simulink model "sampleModel162"  (Simulink 9.1)
settings: Solver=VariableStepAuto  StartTime=0.0  StopTime=10.0  RelTol=1e-3
undefined symbols (not defined in the file): DiscIntNeverNeededParam, magnitude, Newton, Raphson
libraries: simulink x49
(part 1 of 2)
settings Model: SuppressorTable="22 serialization::archive 11 0 6 0 0 2 8 0 0 0 0 6 0 0 1 0 22 sampleModel162/cfblk89 0 6 0 0 2 8 0 0 0 0 6 41 Simulink:DataType:WarningOverFlowDetected 0 0 0 6 0  0  0 0 0 0 8 20160608 0 0 0 15 23 17 0 1 40 SimulinkFixedPoint:util:Overflowoccurred 0 0 0  0  8 20160608 0 15 23 17 0 1 1 0 22 sampleModel162/cfblk90 2 8 0 41 Simulink:DataType:WarningOverFlowDetected 0 0 0  0  8 20160608 0 15 23 17 0 1 40 SimulinkFixedPoint:util:Overflowoccurred 0 0 0  0  8 20160608 0 15 23 17 0 1"  Creator=DELL  LastModifiedBy=DELL
settings DataIOCC: SaveFormat=Dataset
settings OptimizationCC: LifeSpan=auto
settings DebuggingCC: UnderspecifiedInitializationDetection=Simplified  MergeDetectMultiDrivingBlocksExec=error  SFUnexpectedBacktrackingDiag=error  SFNoUnconditionalDefaultTransitionDiag=error  SFExecutionAtInitializationDiag=warning
settings HardwareCC: ProdBitPerPointer=64  ProdBitPerSizeT=64  ProdBitPerPtrDiffT=64  ProdLargestAtomicFloat=Float  ProdIntDivRoundTo=Zero  ProdEndianess=LittleEndian  ProdWordSize=64  ProdHWDeviceType=Intel->x86-64 (Windows64)
settings ModelReferenceCC: PropagateSignalLabelsOutOfModel=on
settings CodeAppCC: StateflowObjectComments=off
settings GRTTargetCC: TargetLangStandard=C99 (ISO)  CombineOutputUpdateFcns=on  GRTInterface=off
settings ConfigComp: CovMetricSettings=dwe  CovHtmlReporting=off  CovSaveCumulativeToWorkspaceVar=off  CovSaveSingleToWorkspaceVar=off  CovExternalEMLEnable=on

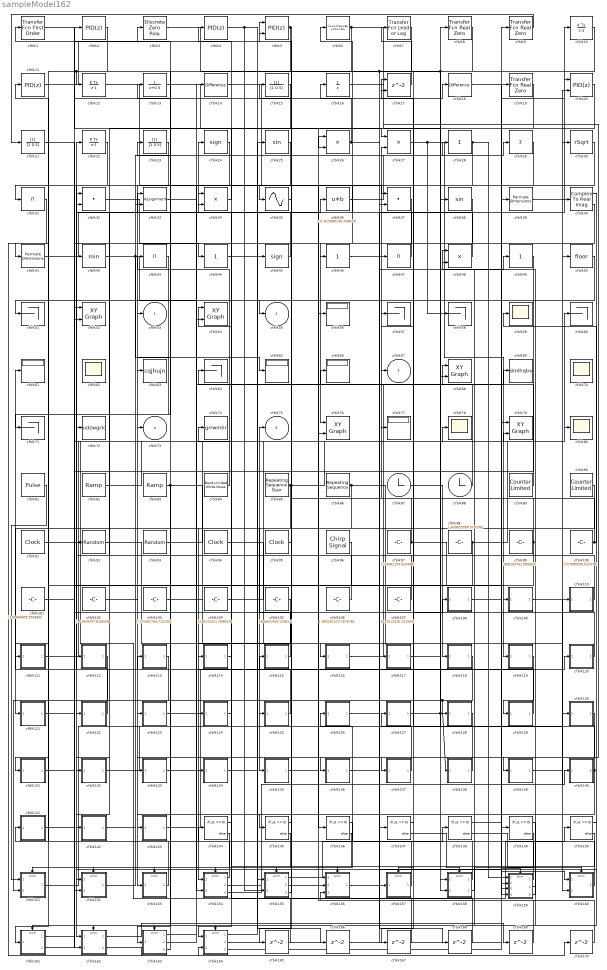
== system sampleModel162 ==
  cfblk1 : simulink/Discrete/Transfer Fcn First Order  PoleZ=0.95  ICPrevOutput=0.0  DoSatur=off
      settings: SourceProductName=Simulink
  cfblk10 : DiscreteIntegrator  ICPrevOutput=DiscIntNeverNeededParam  ICPrevScaledInput=DiscIntNeverNeededParam
  cfblk100 : Constant  Value=[727898558.012478]  SampleTime=1
  cfblk101 : Constant  Value=[149946805.550680]  SampleTime=1
  cfblk102 : Constant  Value=[-62429797.816093]  SampleTime=1
  cfblk103 : Constant  Value=[-175382764.712235]  SampleTime=1
  cfblk104 : Constant  Value=[146113221.789037]  SampleTime=1
  cfblk105 : Constant  Value=[906421434.125611]  SampleTime=1
  cfblk106 : Constant  Value=[-865261573.767678]  SampleTime=1
  cfblk107 : Constant  Value=[813312335.221064]  SampleTime=1
  cfblk108 : Subsystem
  cfblk109 : Subsystem
  cfblk11 : simulink/Continuous/PID Controller  Controller=PID  TimeDomain=Discrete-time  SampleTime=1  IntegratorMethod=Forward Euler  FilterMethod=Forward Euler  Form=Parallel  UseFilter=on  ControllerParametersSource=internal  P=1  I=1  D=0  N=100  InitialConditionSource=internal  InitialConditionForIntegrator=0  InitialConditionForFilter=0  ExternalReset=none  LimitOutput=off  UpperSaturationLimit=inf  LowerSaturationLimit=-inf  LinearizeAsGain=off  AntiWindupMode=none  Kb=1  TrackingMode=off  Kt=1  PParamMin=[]  PParamMax=[]  IParamMin=[]  IParamMax=[]  DParamMin=[]  DParamMax=[]  NParamMin=[]  NParamMax=[]  KbParamMin=[]  KbParamMax=[]  KtParamMin=[]  KtParamMax=[]  POutMin=[]  POutMax=[]  IOutMin=[]  IOutMax=[]  DOutMin=[]  DOutMax=[]  NOutMin=[]  NOutMax=[]  KbOutMin=[]  KbOutMax=[]  KtOutMin=[]  KtOutMax=[]  IntegratorOutMin=[]  IntegratorOutMax=[]  FilterOutMin=[]  FilterOutMax=[]  SumOutMin=[]  SumOutMax=[]  SumI1OutMin=[]  SumI1OutMax=[]  SumI2OutMin=[]  SumI2OutMax=[]  SumI3OutMin=[]  SumI3OutMax=[]  SumDOutMin=[]  SumDOutMax=[]  SaturationOutMin=[]  SaturationOutMax=[]  IntegratorContinuousStateAttributes=''  IntegratorStateMustResolveToSignalObject=off  IntegratorRTWStateStorageClass=Auto  FilterContinuousStateAttributes=''  FilterStateMustResolveToSignalObject=off  FilterRTWStateStorageClass=Auto  DifferentiatorICPrevScaledInput=0  DifferentiatorOutMin=[]  DifferentiatorOutMax=[]  FilterDiffOutCoefMin=[]  FilterDiffOutCoefMax=[]  SumDenOutMin=[]  SumDenOutMax=[]  SumNumOutMin=[]  SumNumOutMax=[]  ReciprocalOutMin=[]  ReciprocalOutMax=[]  DivideOutMin=[]  DivideOutMax=[]  TunerSelectOption=Transfer Function Based (PID Tuner App)
  cfblk110 : Subsystem
  cfblk111 : Subsystem
  cfblk112 : Subsystem
  cfblk113 : Subsystem
  cfblk114 : Subsystem
  cfblk115 : Subsystem
  cfblk116 : Subsystem
  cfblk117 : Subsystem
  cfblk118 : Subsystem
  cfblk119 : Subsystem
  cfblk12 : DiscreteIntegrator  ICPrevOutput=DiscIntNeverNeededParam  ICPrevScaledInput=DiscIntNeverNeededParam
  cfblk120 : Subsystem
  cfblk121 : Subsystem
  cfblk122 : Subsystem
  cfblk123 : Subsystem
  cfblk124 : Subsystem
  cfblk125 : Subsystem
  cfblk126 : Subsystem
  cfblk127 : Subsystem
  cfblk128 : Subsystem
  cfblk129 : Subsystem
  cfblk13 : DiscreteTransferFcn  SampleTime=1
  cfblk130 : Subsystem
  cfblk131 : Subsystem
  cfblk132 : Subsystem
  cfblk133 : Subsystem
  cfblk134 : Subsystem
  cfblk135 : Subsystem
  cfblk136 : Subsystem
  cfblk137 : Subsystem
  cfblk138 : Subsystem
  cfblk139 : Subsystem
  cfblk14 : simulink/Discrete/Difference  ICPrevInput=0.0  OutMin=[]  OutMax=[]  OutDataTypeStr=Inherit: Inherit via back propagation  OutDataType=fixdt(1, 16)  OutScaling=2^-10  DoSatur=off
  cfblk140 : Subsystem
  cfblk141 : Subsystem
  cfblk142 : Subsystem
  cfblk143 : Subsystem
  cfblk{144..150} (7 alike) : If  IfExpression=u1 >= 0  SampleTime=1
  cfblk15 : DiscreteFilter  SampleTime=1
  cfblk151 : Subsystem  TreatAsAtomicUnit=on
  cfblk152 : Subsystem  TreatAsAtomicUnit=on
  cfblk153 : Subsystem  TreatAsAtomicUnit=on
  cfblk154 : Subsystem  TreatAsAtomicUnit=on
  cfblk155 : Subsystem  TreatAsAtomicUnit=on
  cfblk156 : Subsystem  TreatAsAtomicUnit=on
  cfblk157 : Subsystem  TreatAsAtomicUnit=on
  cfblk158 : Subsystem  TreatAsAtomicUnit=on
  cfblk159 : Subsystem  TreatAsAtomicUnit=on
  cfblk16 : UnitDelay
  cfblk160 : Subsystem  TreatAsAtomicUnit=on
  cfblk161 : Subsystem  TreatAsAtomicUnit=on
  cfblk162 : Subsystem  TreatAsAtomicUnit=on
  cfblk163 : Subsystem  TreatAsAtomicUnit=on
  cfblk164 : Subsystem  TreatAsAtomicUnit=on
  cfblk{165..170} (6 alike) : Delay  SampleTime=1
  cfblk17 : Delay  ShowEnablePort=on  SampleTime=1
      settings: InputPortMap=u0,e6
  cfblk18 : simulink/Discrete/Difference  ICPrevInput=0.0  OutMin=[]  OutMax=[]  OutDataTypeStr=Inherit: Inherit via back propagation  OutDataType=fixdt(1, 16)  OutScaling=2^-10  DoSatur=off
  cfblk19 : simulink/Discrete/Transfer Fcn Real Zero  ZeroZ=0.75  ICPrevInput=0.0  DoSatur=off
      settings: SourceProductName=Simulink  SourceProductBaseCode=SL
  cfblk2 : simulink/Continuous/PID Controller  Controller=PID  TimeDomain=Discrete-time  SampleTime=1  IntegratorMethod=Forward Euler  FilterMethod=Forward Euler  Form=Parallel  UseFilter=on  ControllerParametersSource=internal  P=1  I=1  D=0  N=100  InitialConditionSource=internal  InitialConditionForIntegrator=0  InitialConditionForFilter=0  ExternalReset=none  LimitOutput=off  UpperSaturationLimit=inf  LowerSaturationLimit=-inf  LinearizeAsGain=off  AntiWindupMode=none  Kb=1  TrackingMode=off  Kt=1  PParamMin=[]  PParamMax=[]  IParamMin=[]  IParamMax=[]  DParamMin=[]  DParamMax=[]  NParamMin=[]  NParamMax=[]  KbParamMin=[]  KbParamMax=[]  KtParamMin=[]  KtParamMax=[]  POutMin=[]  POutMax=[]  IOutMin=[]  IOutMax=[]  DOutMin=[]  DOutMax=[]  NOutMin=[]  NOutMax=[]  KbOutMin=[]  KbOutMax=[]  KtOutMin=[]  KtOutMax=[]  IntegratorOutMin=[]  IntegratorOutMax=[]  FilterOutMin=[]  FilterOutMax=[]  SumOutMin=[]  SumOutMax=[]  SumI1OutMin=[]  SumI1OutMax=[]  SumI2OutMin=[]  SumI2OutMax=[]  SumI3OutMin=[]  SumI3OutMax=[]  SumDOutMin=[]  SumDOutMax=[]  SaturationOutMin=[]  SaturationOutMax=[]  IntegratorContinuousStateAttributes=''  IntegratorStateMustResolveToSignalObject=off  IntegratorRTWStateStorageClass=Auto  FilterContinuousStateAttributes=''  FilterStateMustResolveToSignalObject=off  FilterRTWStateStorageClass=Auto  DifferentiatorICPrevScaledInput=0  DifferentiatorOutMin=[]  DifferentiatorOutMax=[]  FilterDiffOutCoefMin=[]  FilterDiffOutCoefMax=[]  SumDenOutMin=[]  SumDenOutMax=[]  SumNumOutMin=[]  SumNumOutMax=[]  ReciprocalOutMin=[]  ReciprocalOutMax=[]  DivideOutMin=[]  DivideOutMax=[]  TunerSelectOption=Transfer Function Based (PID Tuner App)
  cfblk20 : simulink/Continuous/PID Controller (2DOF)  Controller=PID  TimeDomain=Discrete-time  SampleTime=1  IntegratorMethod=Forward Euler  FilterMethod=Forward Euler  Form=Parallel  UseFilter=on  ControllerParametersSource=internal  P=1  I=1  D=0  N=100  b=1  c=1  InitialConditionSource=internal  InitialConditionForIntegrator=0  InitialConditionForFilter=0  ExternalReset=none  LimitOutput=off  UpperSaturationLimit=inf  LowerSaturationLimit=-inf  LinearizeAsGain=off  AntiWindupMode=none  Kb=1  TrackingMode=off  Kt=1  PParamMin=[]  PParamMax=[]  IParamMin=[]  IParamMax=[]  DParamMin=[]  DParamMax=[]  NParamMin=[]  NParamMax=[]  bParamMin=[]  bParamMax=[]  cParamMin=[]  cParamMax=[]  KbParamMin=[]  KbParamMax=[]  KtParamMin=[]  KtParamMax=[]  POutMin=[]  POutMax=[]  IOutMin=[]  IOutMax=[]  DOutMin=[]  DOutMax=[]  NOutMin=[]  NOutMax=[]  bOutMin=[]  bOutMax=[]  cOutMin=[]  cOutMax=[]  KbOutMin=[]  KbOutMax=[]  KtOutMin=[]  KtOutMax=[]  IntegratorOutMin=[]  IntegratorOutMax=[]  FilterOutMin=[]  FilterOutMax=[]  SumOutMin=[]  SumOutMax=[]  Sum1OutMin=[]  Sum1OutMax=[]  Sum2OutMin=[]  Sum2OutMax=[]  Sum3OutMin=[]  Sum3OutMax=[]  SumI1OutMin=[]  SumI1OutMax=[]  SumI2OutMin=[]  SumI2OutMax=[]  SumI3OutMin=[]  SumI3OutMax=[]  SumDOutMin=[]  SumDOutMax=[]  SaturationOutMin=[]  SaturationOutMax=[]  IntegratorContinuousStateAttributes=''  IntegratorStateMustResolveToSignalObject=off  IntegratorRTWStateStorageClass=Auto  FilterContinuousStateAttributes=''  FilterStateMustResolveToSignalObject=off  FilterRTWStateStorageClass=Auto  DifferentiatorICPrevScaledInput=0  DifferentiatorOutMin=[]  DifferentiatorOutMax=[]  FilterDiffOutCoefMin=[]  FilterDiffOutCoefMax=[]  SumDenOutMin=[]  SumDenOutMax=[]  SumNumOutMin=[]  SumNumOutMax=[]  ReciprocalOutMin=[]  ReciprocalOutMax=[]  DivideOutMin=[]  DivideOutMax=[]  TunerSelectOption=Transfer Function Based (PID Tuner App)
  cfblk21 : DiscreteFilter  SampleTime=1
  cfblk22 : DiscreteIntegrator  ICPrevOutput=DiscIntNeverNeededParam  ICPrevScaledInput=DiscIntNeverNeededParam
  cfblk23 : DiscreteFilter  SampleTime=1
  cfblk24 : Signum
  cfblk25 : Trigonometry
  cfblk26 : Product  Inputs=**
  cfblk27 : Product
  cfblk{28,44,46,49} (4 alike) : simulink/Math Operations/Slider Gain  gain=1  low=0  high=2
  cfblk29 : Sum  Inputs=+
  cfblk3 : DiscreteZeroPole  Poles=[0 0.5]  Gain=1
  cfblk30 : Sqrt  Operator=rSqrt  AlgorithmType=Newton-Raphson  SaturateOnIntegerOverflow=on
  cfblk31 : Product  Inputs=*
  cfblk32 : DotProduct  InputSameDT=on  OutDataTypeStr=Inherit: Inherit via internal rule
  cfblk33 : Assignment  DiagnosticForDimensions=Warning  IndexOptions=Index vector (dialog)  Indices=1  OutputSizes=1
  cfblk34 : Product  Inputs=**
  cfblk35 : Sin  TimeSource=Use external signal  SampleTime=0
  cfblk36 : Bias  Bias=[-815080136.708875]
  cfblk37 : DotProduct  InputSameDT=on  OutDataTypeStr=Inherit: Inherit via internal rule
  cfblk38 : Trigonometry
  cfblk39 : PermuteDimensions
  cfblk4 : simulink/Continuous/PID Controller  Controller=PID  TimeDomain=Discrete-time  SampleTime=1  IntegratorMethod=Forward Euler  FilterMethod=Forward Euler  Form=Parallel  UseFilter=on  ControllerParametersSource=internal  P=1  I=1  D=0  N=100  InitialConditionSource=internal  InitialConditionForIntegrator=0  InitialConditionForFilter=0  ExternalReset=none  LimitOutput=off  UpperSaturationLimit=inf  LowerSaturationLimit=-inf  LinearizeAsGain=off  AntiWindupMode=none  Kb=1  TrackingMode=off  Kt=1  PParamMin=[]  PParamMax=[]  IParamMin=[]  IParamMax=[]  DParamMin=[]  DParamMax=[]  NParamMin=[]  NParamMax=[]  KbParamMin=[]  KbParamMax=[]  KtParamMin=[]  KtParamMax=[]  POutMin=[]  POutMax=[]  IOutMin=[]  IOutMax=[]  DOutMin=[]  DOutMax=[]  NOutMin=[]  NOutMax=[]  KbOutMin=[]  KbOutMax=[]  KtOutMin=[]  KtOutMax=[]  IntegratorOutMin=[]  IntegratorOutMax=[]  FilterOutMin=[]  FilterOutMax=[]  SumOutMin=[]  SumOutMax=[]  SumI1OutMin=[]  SumI1OutMax=[]  SumI2OutMin=[]  SumI2OutMax=[]  SumI3OutMin=[]  SumI3OutMax=[]  SumDOutMin=[]  SumDOutMax=[]  SaturationOutMin=[]  SaturationOutMax=[]  IntegratorContinuousStateAttributes=''  IntegratorStateMustResolveToSignalObject=off  IntegratorRTWStateStorageClass=Auto  FilterContinuousStateAttributes=''  FilterStateMustResolveToSignalObject=off  FilterRTWStateStorageClass=Auto  DifferentiatorICPrevScaledInput=0  DifferentiatorOutMin=[]  DifferentiatorOutMax=[]  FilterDiffOutCoefMin=[]  FilterDiffOutCoefMax=[]  SumDenOutMin=[]  SumDenOutMax=[]  SumNumOutMin=[]  SumNumOutMax=[]  ReciprocalOutMin=[]  ReciprocalOutMax=[]  DivideOutMin=[]  DivideOutMax=[]  TunerSelectOption=Transfer Function Based (PID Tuner App)
  cfblk40 : ComplexToRealImag
  cfblk41 : PermuteDimensions
  cfblk42 : MinMax
  cfblk43 : Product  Inputs=*
  cfblk45 : Signum
  cfblk47 : Product  Inputs=*
  cfblk48 : Product
  cfblk5 : simulink/Continuous/PID Controller (2DOF)  Controller=PID  TimeDomain=Discrete-time  SampleTime=1  IntegratorMethod=Forward Euler  FilterMethod=Forward Euler  Form=Parallel  UseFilter=on  ControllerParametersSource=internal  P=1  I=1  D=0  N=100  b=1  c=1  InitialConditionSource=internal  InitialConditionForIntegrator=0  InitialConditionForFilter=0  ExternalReset=none  LimitOutput=off  UpperSaturationLimit=inf  LowerSaturationLimit=-inf  LinearizeAsGain=off  AntiWindupMode=none  Kb=1  TrackingMode=off  Kt=1  PParamMin=[]  PParamMax=[]  IParamMin=[]  IParamMax=[]  DParamMin=[]  DParamMax=[]  NParamMin=[]  NParamMax=[]  bParamMin=[]  bParamMax=[]  cParamMin=[]  cParamMax=[]  KbParamMin=[]  KbParamMax=[]  KtParamMin=[]  KtParamMax=[]  POutMin=[]  POutMax=[]  IOutMin=[]  IOutMax=[]  DOutMin=[]  DOutMax=[]  NOutMin=[]  NOutMax=[]  bOutMin=[]  bOutMax=[]  cOutMin=[]  cOutMax=[]  KbOutMin=[]  KbOutMax=[]  KtOutMin=[]  KtOutMax=[]  IntegratorOutMin=[]  IntegratorOutMax=[]  FilterOutMin=[]  FilterOutMax=[]  SumOutMin=[]  SumOutMax=[]  Sum1OutMin=[]  Sum1OutMax=[]  Sum2OutMin=[]  Sum2OutMax=[]  Sum3OutMin=[]  Sum3OutMax=[]  SumI1OutMin=[]  SumI1OutMax=[]  SumI2OutMin=[]  SumI2OutMax=[]  SumI3OutMin=[]  SumI3OutMax=[]  SumDOutMin=[]  SumDOutMax=[]  SaturationOutMin=[]  SaturationOutMax=[]  IntegratorContinuousStateAttributes=''  IntegratorStateMustResolveToSignalObject=off  IntegratorRTWStateStorageClass=Auto  FilterContinuousStateAttributes=''  FilterStateMustResolveToSignalObject=off  FilterRTWStateStorageClass=Auto  DifferentiatorICPrevScaledInput=0  DifferentiatorOutMin=[]  DifferentiatorOutMax=[]  FilterDiffOutCoefMin=[]  FilterDiffOutCoefMax=[]  SumDenOutMin=[]  SumDenOutMax=[]  SumNumOutMin=[]  SumNumOutMax=[]  ReciprocalOutMin=[]  ReciprocalOutMax=[]  DivideOutMin=[]  DivideOutMax=[]  TunerSelectOption=Transfer Function Based (PID Tuner App)
  cfblk50 : Rounding
  cfblk{51,57..58,60,64,71} (6 alike) : Terminator
  cfblk{52,54,68,76,79} (5 alike) : simulink/Sinks/XY Graph  xmin=-1  xmax=1  ymin=-1  ymax=1  st=-1
  cfblk{56,61,65..66,77} (5 alike) : Display
  cfblk{59,62,70,78,80} (5 alike) : Scope
      cfblk62 settings: Floating=on
      cfblk70 settings: Floating=on
  cfblk6 : DiscreteStateSpace
  cfblk63 : ToWorkspace  VariableName=cqjhujn  SaveFormat=Timeseries  SampleTime=-1
  cfblk69 : ToWorkspace  VariableName=dmlhqbv  SaveFormat=Timeseries  SampleTime=-1
  cfblk7 : simulink/Discrete/Transfer Fcn Lead or Lag  PoleZ=0.95  ZeroZ=0.75  ICPrevOutput=0.0  ICPrevInput=0.0  DoSatur=off
      settings: SourceProductName=Simulink  SourceProductBaseCode=SL
  cfblk72 : ToWorkspace  VariableName=udzwgck  SaveFormat=Timeseries  SampleTime=-1
  cfblk74 : ToWorkspace  VariableName=grrwmhr  SaveFormat=Timeseries  SampleTime=-1
  cfblk8 : simulink/Discrete/Transfer Fcn Real Zero  ZeroZ=0.75  ICPrevInput=0.0  DoSatur=off
      settings: SourceProductName=Simulink  SourceProductBaseCode=SL
  cfblk81 : DiscretePulseGenerator  PulseType=Time based  Amplitude=[-1371846.449111]  Period=[72395569.989002]  PulseWidth=5  PhaseDelay=[9.000000]
  cfblk82 : simulink/Sources/Ramp  slope=[5140.421484]  start=[47.590381]  InitialOutput=[-206299.463391]
  cfblk83 : simulink/Sources/Ramp  slope=[-8341.390196]  start=[43.939396]  InitialOutput=[-754794.637201]
  cfblk84 : simulink/Sources/Band-Limited White Noise  Cov=[7560464618.662546]  Ts=0.1  seed=[9065001128.000000]
  cfblk85 : simulink/Sources/Repeating Sequence Stair  OutValues=[-79011152.103958, -456733271.397849]  tsamp=-1  OutMin=[]  OutMax=[]  OutDataTypeStr=double  OutputDataTypeScalingMode=double  OutDataType=fixdt(0,8)  ConRadixGroup=Best Precision: Vector-wise  OutScaling=2^-12
  cfblk86 : simulink/Sources/Repeating Sequence  rep_seq_t=[0 2]  rep_seq_y=[-862919646.627076, -121342680.384582]
  cfblk87 : Clock
  cfblk88 : Clock
  cfblk89 : simulink/Sources/Counter Limited  uplimit=[824.000000]  tsamp=-1
  cfblk9 : simulink/Discrete/Transfer Fcn Real Zero  ZeroZ=0.75  ICPrevInput=0.0  DoSatur=off
      settings: SourceProductName=Simulink  SourceProductBaseCode=SL
  cfblk90 : simulink/Sources/Counter Limited  uplimit=[298.000000]  tsamp=-1
  cfblk91 : DigitalClock
  cfblk92 : RandomNumber  Mean=[-60678.124830]  Variance=[62859.906878]  Seed=[18431920.000000]  SampleTime=0.1
  cfblk93 : UniformRandomNumber  Minimum=[-2959977652.124598]  Maximum=[440301292.630647]  Seed=[41048107.000000]  SampleTime=0.1
  cfblk94 : DigitalClock
  cfblk95 : DigitalClock
  cfblk96 : simulink/Sources/Chirp Signal  f1=[-414625876.542801]  T=[476939218.482737]  f2=[-707117522.097986]
  cfblk97 : Constant  Value=[174581154.924498]  SampleTime=1
  cfblk98 : Constant  Value=[-639855958.573706]  SampleTime=1
  cfblk99 : Constant  Value=[965265761.586653]  SampleTime=1
  cfblk53 : Outport
  cfblk55 : Outport  Port=2
  cfblk67 : Outport  Port=3
  cfblk73 : Outport  Port=4
  cfblk75 : Outport  Port=5
  wires:
  cfblk23/1 -> cfblk153/1(cfblk1)
  cfblk84/1 -> cfblk1/1
  cfblk91/1 -> cfblk150/1, cfblk79/2
  cfblk90/1 -> cfblk154/1(cfblk1)
  cfblk114/1(cfblk2) -> cfblk164/1(cfblk1)
  cfblk41/1 -> cfblk33/1
  cfblk155/1(cfblk2) -> cfblk148/1
  cfblk112/1(cfblk2) -> cfblk162/1(cfblk1)
  cfblk11/1 -> cfblk5/1
  cfblk110/1(cfblk2) -> cfblk22/1
  cfblk50/1 -> cfblk51/1
  cfblk116/1(cfblk2) -> cfblk68/1
  cfblk100/1 -> cfblk59/1, cfblk77/1
  cfblk13/1 -> cfblk27/1
  cfblk36/1 -> cfblk29/1
  cfblk6/1 -> cfblk139/1(cfblk1), cfblk35/1
  cfblk24/1 -> cfblk63/1
  cfblk115/1(cfblk2) -> cfblk75/1
  cfblk94/1 -> cfblk116/1(cfblk1)
  cfblk48/1 -> cfblk24/1
  cfblk86/1 -> cfblk121/1(cfblk1), cfblk158/2(cfblk16)
  cfblk119/1(cfblk2) -> cfblk129/1(cfblk1)
  cfblk25/1 -> cfblk122/1(cfblk1)
  cfblk39/1 -> cfblk10/1
  cfblk140/1(cfblk2) -> cfblk143/1(cfblk1), cfblk17/2
  cfblk105/1 -> cfblk114/1(cfblk1)
  cfblk12/1 -> cfblk146/1
  cfblk81/1 -> cfblk151/1(cfblk1)
  cfblk82/1 -> cfblk14/1
  cfblk129/1(cfblk2) -> cfblk61/1
  cfblk99/1 -> cfblk27/2, cfblk131/1(cfblk1)
  cfblk38/1 -> cfblk76/1
  cfblk85/1 -> cfblk145/1, cfblk47/1, cfblk135/1(cfblk1)
  cfblk20/1 -> cfblk73/1
  cfblk122/1(cfblk2) -> cfblk72/1
  cfblk101/1 -> cfblk2/1
  cfblk14/1 -> cfblk37/1
  cfblk27/1 -> cfblk119/1(cfblk1), cfblk58/1
  cfblk37/1 -> cfblk42/1
  cfblk102/1 -> cfblk123/1(cfblk1)
  cfblk10/1 -> cfblk137/1(cfblk1), cfblk68/2
  cfblk160/1(cfblk2) -> cfblk126/1(cfblk1)
  cfblk133/1(cfblk2) -> cfblk26/1
  cfblk43/1 -> cfblk71/1
  cfblk26/1 -> cfblk16/1, cfblk159/2(cfblk8)
  cfblk97/1 -> cfblk149/1, cfblk5/2
  cfblk123/1(cfblk2) -> cfblk120/1(cfblk1)
  cfblk151/1(cfblk2) -> cfblk110/1(cfblk1)
  cfblk44/1 -> cfblk45/1
  cfblk87/1 -> cfblk118/1(cfblk1)
  cfblk21/1 -> cfblk109/1(cfblk1)
  cfblk4/1 -> cfblk155/2(cfblk14), cfblk166/1
  cfblk135/1(cfblk2) -> cfblk56/1
  cfblk98/1 -> cfblk60/1, cfblk134/1(cfblk1)
  cfblk88/1 -> cfblk64/1
  cfblk152/1(cfblk2) -> cfblk36/1
  cfblk89/1 -> cfblk67/1
  cfblk158/1(cfblk2) -> cfblk34/1
  cfblk153/1(cfblk2) -> cfblk141/1(cfblk1)
  cfblk96/1 -> cfblk161/1(cfblk1)
  cfblk103/1 -> cfblk157/1(cfblk1)
  cfblk8/1 -> cfblk37/2, cfblk125/1(cfblk1)
  cfblk95/1 -> cfblk15/1
  cfblk93/1 -> cfblk19/1
  cfblk113/1(cfblk2) -> cfblk132/1(cfblk1)
  cfblk137/1(cfblk2) -> cfblk127/1(cfblk1)
  cfblk15/1 -> cfblk124/1(cfblk1)
  cfblk29/1 -> cfblk154/2(cfblk7)
  cfblk32/1 -> cfblk44/1
  cfblk134/1(cfblk2) -> cfblk69/1
  cfblk124/1(cfblk2) -> cfblk54/1
  cfblk138/1(cfblk2) -> cfblk136/1(cfblk1)
  cfblk49/1 -> cfblk162/2(cfblk12)
  cfblk121/1(cfblk2) -> cfblk78/1
  cfblk163/1(cfblk2) -> cfblk66/1
  cfblk42/1 -> cfblk54/2, cfblk65/1
  cfblk30/1 -> cfblk46/1
  cfblk19/1 -> cfblk142/1(cfblk1)
  cfblk161/1(cfblk2) -> cfblk108/1(cfblk1)
  cfblk120/1(cfblk2) -> cfblk57/1
  cfblk9/1 -> cfblk21/1
  cfblk28/1 -> cfblk111/1(cfblk1), cfblk159/1(cfblk1)
  cfblk142/1(cfblk2) -> cfblk28/1
  cfblk7/1 -> cfblk31/1
  cfblk3/1 -> cfblk38/1
  cfblk108/1(cfblk2) -> cfblk20/1
  cfblk33/1 -> cfblk17/1
  cfblk136/1(cfblk2) -> cfblk49/1
  cfblk117/1(cfblk2) -> cfblk80/1
  cfblk118/1(cfblk2) -> cfblk151/2(cfblk14), cfblk128/1(cfblk1)
  cfblk31/1 -> cfblk164/2(cfblk10)
  cfblk154/1(cfblk2) -> cfblk113/1(cfblk1)
  cfblk47/1 -> cfblk6/1
  cfblk35/1 -> cfblk55/1
  cfblk132/1(cfblk2) -> cfblk9/1
  cfblk104/1 -> cfblk30/1
  cfblk45/1 -> cfblk23/1
  cfblk143/1(cfblk2) -> cfblk8/1
  cfblk141/1(cfblk2) -> cfblk3/1
  cfblk157/1(cfblk2) -> cfblk11/1
  cfblk109/1(cfblk2) -> cfblk130/1(cfblk1)
  cfblk156/1(cfblk2) -> cfblk40/1
  cfblk106/1 -> cfblk13/1
  cfblk127/1(cfblk2) -> cfblk138/1(cfblk1), cfblk159/3(cfblk9)
  cfblk1/1 -> cfblk26/2
  cfblk17/1 -> cfblk7/1
  cfblk128/1(cfblk2) -> cfblk163/1(cfblk1)
  cfblk161/2(cfblk8) -> cfblk52/1
  cfblk164/1(cfblk2) -> cfblk25/1
  cfblk34/1 -> cfblk4/1
  cfblk2/1 -> cfblk12/1, cfblk41/1
  cfblk5/1 -> cfblk53/1, cfblk165/1
  cfblk154/2(cfblk8) -> cfblk50/1
  cfblk164/2(cfblk11) -> cfblk79/1
  cfblk155/2(cfblk15) -> cfblk140/1(cfblk1)
  cfblk83/1 -> cfblk133/1(cfblk1), cfblk159/4(cfblk10)
  cfblk131/1(cfblk2) -> cfblk18/1
  cfblk154/3(cfblk9) -> cfblk76/2
  cfblk40/1 -> cfblk152/1(cfblk1)
  cfblk18/1 -> cfblk160/1(cfblk1)
  cfblk92/1 -> cfblk160/2(cfblk8)
  cfblk158/2(cfblk17) -> cfblk48/1
  cfblk16/1 -> cfblk158/1(cfblk1)
  cfblk164/3(cfblk12) -> cfblk39/1
  cfblk40/2 -> cfblk152/2(cfblk8)
  cfblk155/3(cfblk16) -> cfblk32/1
  cfblk107/1 -> cfblk32/2
  cfblk46/1 -> cfblk117/1(cfblk1)
  cfblk22/1 -> cfblk52/2
  cfblk139/1(cfblk2) -> cfblk20/2
  cfblk163/2(cfblk6) -> cfblk115/1(cfblk1)
  cfblk111/1(cfblk2) -> cfblk33/2
  cfblk125/1(cfblk2) -> cfblk112/1(cfblk1)
  cfblk159/1(cfblk2) -> cfblk74/1
  cfblk159/2(cfblk11) -> cfblk48/2
  cfblk159/3(cfblk12) -> cfblk144/1
  cfblk163/3(cfblk7) -> cfblk43/1
  cfblk144/1 -> cfblk151/Action
  cfblk144/2 -> cfblk152/Action
  cfblk145/1 -> cfblk153/Action
  cfblk145/2 -> cfblk154/Action
  cfblk146/1 -> cfblk155/Action
  cfblk146/2 -> cfblk156/Action
  cfblk147/1 -> cfblk157/Action
  cfblk147/2 -> cfblk158/Action
  cfblk148/1 -> cfblk159/Action
  cfblk148/2 -> cfblk160/Action
  cfblk149/1 -> cfblk161/Action
  cfblk149/2 -> cfblk162/Action
  cfblk150/1 -> cfblk163/Action
  cfblk150/2 -> cfblk164/Action
  cfblk165/1 -> cfblk34/2
  cfblk166/1 -> cfblk147/1
  cfblk130/1(cfblk2) -> cfblk167/1
  cfblk167/1 -> cfblk155/1(cfblk1)
  cfblk126/1(cfblk2) -> cfblk168/1
  cfblk168/1 -> cfblk156/1(cfblk1)
  cfblk162/1(cfblk2) -> cfblk169/1
  cfblk169/1 -> cfblk156/2(cfblk7)
  cfblk162/2(cfblk13) -> cfblk170/1
  cfblk170/1 -> cfblk156/3(cfblk8)

== system sampleModel162/cfblk108 ==
  cfblk1 : Inport
  cfblk2 : Outport
  wires:
  cfblk1/1 -> cfblk2/1

== system sampleModel162/cfblk109 ==
  cfblk1 : Inport
  cfblk2 : Outport
  wires:
  cfblk1/1 -> cfblk2/1

== system sampleModel162/cfblk110 ==
  cfblk1 : Inport
  cfblk2 : Outport
  wires:
  cfblk1/1 -> cfblk2/1

== system sampleModel162/cfblk111 ==
  cfblk1 : Inport
  cfblk2 : Outport
  wires:
  cfblk1/1 -> cfblk2/1

== system sampleModel162/cfblk112 ==
  cfblk1 : Inport
  cfblk2 : Outport
  wires:
  cfblk1/1 -> cfblk2/1

== system sampleModel162/cfblk113 ==
  cfblk1 : Inport
  cfblk2 : Outport
  wires:
  cfblk1/1 -> cfblk2/1

== system sampleModel162/cfblk114 ==
  cfblk1 : Inport
  cfblk2 : Outport
  wires:
  cfblk1/1 -> cfblk2/1

== system sampleModel162/cfblk115 ==
  cfblk1 : Inport
  cfblk2 : Outport
  wires:
  cfblk1/1 -> cfblk2/1

== system sampleModel162/cfblk116 ==
  cfblk1 : Inport
  cfblk2 : Outport
  wires:
  cfblk1/1 -> cfblk2/1

== system sampleModel162/cfblk117 ==
  cfblk1 : Inport
  cfblk2 : Outport
  wires:
  cfblk1/1 -> cfblk2/1

== system sampleModel162/cfblk118 ==
  cfblk1 : Inport
  cfblk2 : Outport
  wires:
  cfblk1/1 -> cfblk2/1

== system sampleModel162/cfblk119 ==
  cfblk1 : Inport
  cfblk2 : Outport
  wires:
  cfblk1/1 -> cfblk2/1

== system sampleModel162/cfblk120 ==
  cfblk1 : Inport
  cfblk2 : Outport
  wires:
  cfblk1/1 -> cfblk2/1

== system sampleModel162/cfblk121 ==
  cfblk1 : Inport
  cfblk2 : Outport
  wires:
  cfblk1/1 -> cfblk2/1

== system sampleModel162/cfblk122 ==
  cfblk1 : Inport
  cfblk2 : Outport
  wires:
  cfblk1/1 -> cfblk2/1

== system sampleModel162/cfblk123 ==
  cfblk1 : Inport
  cfblk2 : Outport
  wires:
  cfblk1/1 -> cfblk2/1

== system sampleModel162/cfblk124 ==
  cfblk1 : Inport
  cfblk2 : Outport
  wires:
  cfblk1/1 -> cfblk2/1

== system sampleModel162/cfblk125 ==
  cfblk1 : Inport
  cfblk2 : Outport
  wires:
  cfblk1/1 -> cfblk2/1

== system sampleModel162/cfblk126 ==
  cfblk1 : Inport
  cfblk2 : Outport
  wires:
  cfblk1/1 -> cfblk2/1

== system sampleModel162/cfblk127 ==
  cfblk1 : Inport
  cfblk2 : Outport
  wires:
  cfblk1/1 -> cfblk2/1

== system sampleModel162/cfblk128 ==
  cfblk1 : Inport
  cfblk2 : Outport
  wires:
  cfblk1/1 -> cfblk2/1

== system sampleModel162/cfblk129 ==
  cfblk1 : Inport
  cfblk2 : Outport
  wires:
  cfblk1/1 -> cfblk2/1

== system sampleModel162/cfblk130 ==
  cfblk1 : Inport
  cfblk2 : Outport
  wires:
  cfblk1/1 -> cfblk2/1

== system sampleModel162/cfblk131 ==
  cfblk1 : Inport
  cfblk2 : Outport
  wires:
  cfblk1/1 -> cfblk2/1

== system sampleModel162/cfblk132 ==
  cfblk1 : Inport
  cfblk2 : Outport
  wires:
  cfblk1/1 -> cfblk2/1

== system sampleModel162/cfblk133 ==
  cfblk1 : Inport
  cfblk2 : Outport
  wires:
  cfblk1/1 -> cfblk2/1

== system sampleModel162/cfblk134 ==
  cfblk1 : Inport
  cfblk2 : Outport
  wires:
  cfblk1/1 -> cfblk2/1

== system sampleModel162/cfblk135 ==
  cfblk1 : Inport
  cfblk2 : Outport
  wires:
  cfblk1/1 -> cfblk2/1

== system sampleModel162/cfblk136 ==
  cfblk1 : Inport
  cfblk2 : Outport
  wires:
  cfblk1/1 -> cfblk2/1

== system sampleModel162/cfblk137 ==
  cfblk1 : Inport
  cfblk2 : Outport
  wires:
  cfblk1/1 -> cfblk2/1

== system sampleModel162/cfblk138 ==
  cfblk1 : Inport
  cfblk2 : Outport
  wires:
  cfblk1/1 -> cfblk2/1

== system sampleModel162/cfblk139 ==
  cfblk1 : Inport
  cfblk2 : Outport
  wires:
  cfblk1/1 -> cfblk2/1

== system sampleModel162/cfblk140 ==
  cfblk1 : Inport
  cfblk2 : Outport
  wires:
  cfblk1/1 -> cfblk2/1

== system sampleModel162/cfblk141 ==
  cfblk1 : Inport
  cfblk2 : Outport
  wires:
  cfblk1/1 -> cfblk2/1

== system sampleModel162/cfblk142 ==
  cfblk1 : Inport
  cfblk2 : Outport
  wires:
  cfblk1/1 -> cfblk2/1

== system sampleModel162/cfblk143 ==
  cfblk1 : Inport
  cfblk2 : Outport
  wires:
  cfblk1/1 -> cfblk2/1

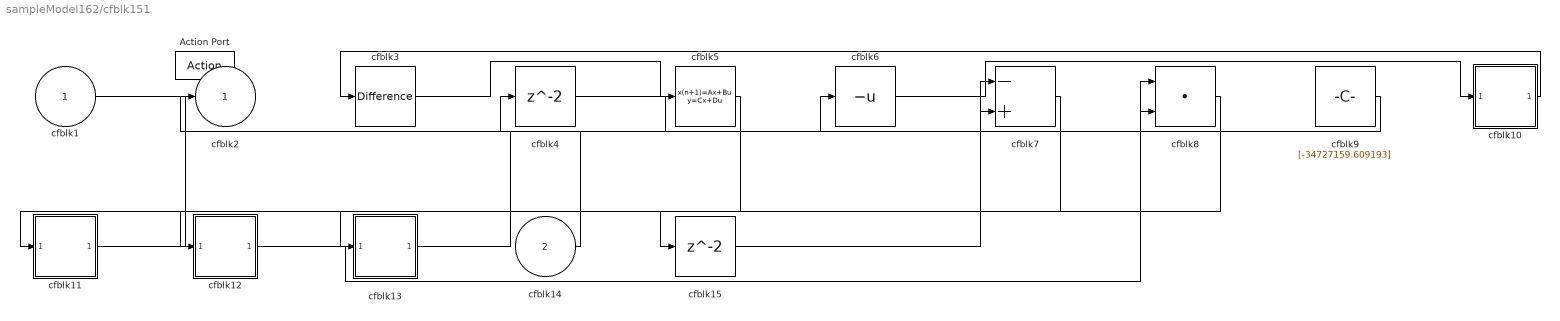
== system sampleModel162/cfblk151 ==
  cfblk1 : Inport
  cfblk14 : Inport  Port=2
  Action Port : ActionPort  ActionType=then
  cfblk10 : Subsystem
  cfblk11 : Subsystem
  cfblk12 : Subsystem
  cfblk13 : Subsystem
  cfblk15 : Delay
  cfblk3 : simulink/Discrete/Difference  ICPrevInput=0.0  OutMin=[]  OutMax=[]  OutDataTypeStr=Inherit: Inherit via back propagation  OutDataType=fixdt(1, 16)  OutScaling=2^-10  DoSatur=off
  cfblk4 : Delay
  cfblk5 : DiscreteStateSpace  SampleTime=-1
  cfblk6 : UnaryMinus
  cfblk7 : Sum  Inputs=-+
  cfblk8 : DotProduct  InputSameDT=on  OutDataTypeStr=Inherit: Inherit via internal rule
  cfblk9 : Constant  Value=[-34727159.609193]  SampleTime=1
  cfblk2 : Outport
  wires:
  cfblk5/1 -> cfblk11/1(cfblk1)
  cfblk6/1 -> cfblk10/1(cfblk1)
  cfblk14/1 -> cfblk4/1
  cfblk10/1(cfblk2) -> cfblk3/1
  cfblk12/1(cfblk2) -> cfblk8/1
  cfblk1/1 -> cfblk13/1(cfblk1)
  cfblk13/1(cfblk2) -> cfblk6/1
  cfblk11/1(cfblk2) -> cfblk7/1
  cfblk7/1 -> cfblk12/1(cfblk1)
  cfblk4/1 -> cfblk8/2
  cfblk3/1 -> cfblk5/1
  cfblk9/1 -> cfblk2/1
  cfblk8/1 -> cfblk15/1
  cfblk15/1 -> cfblk7/2

== system sampleModel162/cfblk152 ==
  cfblk1 : Inport
  cfblk8 : Inport  Port=2
  Action Port : ActionPort  ActionType=else
  cfblk3 : DiscreteIntegrator  SampleTime=-1  ICPrevOutput=DiscIntNeverNeededParam  ICPrevScaledInput=DiscIntNeverNeededParam
  cfblk4 : Gain  Gain=[981288571.279234]
  cfblk5 : Constant  Value=[52814938.085575]  SampleTime=1
  cfblk6 : Subsystem
  cfblk7 : Subsystem
  cfblk9 : Delay
  cfblk2 : Outport
  wires:
  cfblk1/1 -> cfblk3/1
  cfblk5/1 -> cfblk2/1
  cfblk4/1 -> cfblk6/1(cfblk1)
  cfblk8/1 -> cfblk7/1(cfblk1)
  cfblk6/1(cfblk2) -> cfblk9/1
  cfblk9/1 -> cfblk4/1

== system sampleModel162/cfblk153 ==
  cfblk1 : Inport
  Action Port : ActionPort  ActionType=then
  cfblk3 : DiscreteZeroPole  Poles=[0 0.5]  Gain=1  SampleTime=-1
  cfblk4 : MinMax  Function=max
  cfblk5 : Sqrt  SaturateOnIntegerOverflow=on
  cfblk6 : Constant  Value=[721223764.128831]  SampleTime=1
  cfblk7 : Constant  Value=[842996176.805068]  SampleTime=1
  cfblk8 : Subsystem
  cfblk9 : Subsystem
  cfblk2 : Outport
  wires:
  cfblk6/1 -> cfblk9/1(cfblk1)
  cfblk9/1(cfblk2) -> cfblk5/1
  cfblk5/1 -> cfblk2/1
  cfblk4/1 -> cfblk8/1(cfblk1)
  cfblk7/1 -> cfblk4/1
  cfblk1/1 -> cfblk3/1

== system sampleModel162/cfblk154 ==
  cfblk1 : Inport
  cfblk7 : Inport  Port=2
  Action Port : ActionPort  ActionType=else
  cfblk10 : DataTypeConversion
  cfblk3 : simulink/Continuous/PID Controller (2DOF)  Controller=PID  TimeDomain=Discrete-time  SampleTime=-1  IntegratorMethod=Forward Euler  FilterMethod=Forward Euler  Form=Parallel  UseFilter=on  ControllerParametersSource=internal  P=1  I=1  D=0  N=100  b=1  c=1  InitialConditionSource=internal  InitialConditionForIntegrator=0  InitialConditionForFilter=0  ExternalReset=none  LimitOutput=off  UpperSaturationLimit=inf  LowerSaturationLimit=-inf  LinearizeAsGain=off  AntiWindupMode=none  Kb=1  TrackingMode=off  Kt=1  PParamMin=[]  PParamMax=[]  IParamMin=[]  IParamMax=[]  DParamMin=[]  DParamMax=[]  NParamMin=[]  NParamMax=[]  bParamMin=[]  bParamMax=[]  cParamMin=[]  cParamMax=[]  KbParamMin=[]  KbParamMax=[]  KtParamMin=[]  KtParamMax=[]  POutMin=[]  POutMax=[]  IOutMin=[]  IOutMax=[]  DOutMin=[]  DOutMax=[]  NOutMin=[]  NOutMax=[]  bOutMin=[]  bOutMax=[]  cOutMin=[]  cOutMax=[]  KbOutMin=[]  KbOutMax=[]  KtOutMin=[]  KtOutMax=[]  IntegratorOutMin=[]  IntegratorOutMax=[]  FilterOutMin=[]  FilterOutMax=[]  SumOutMin=[]  SumOutMax=[]  Sum1OutMin=[]  Sum1OutMax=[]  Sum2OutMin=[]  Sum2OutMax=[]  Sum3OutMin=[]  Sum3OutMax=[]  SumI1OutMin=[]  SumI1OutMax=[]  SumI2OutMin=[]  SumI2OutMax=[]  SumI3OutMin=[]  SumI3OutMax=[]  SumDOutMin=[]  SumDOutMax=[]  SaturationOutMin=[]  SaturationOutMax=[]  IntegratorContinuousStateAttributes=''  IntegratorStateMustResolveToSignalObject=off  IntegratorRTWStateStorageClass=Auto  FilterContinuousStateAttributes=''  FilterStateMustResolveToSignalObject=off  FilterRTWStateStorageClass=Auto  DifferentiatorICPrevScaledInput=0  DifferentiatorOutMin=[]  DifferentiatorOutMax=[]  FilterDiffOutCoefMin=[]  FilterDiffOutCoefMax=[]  SumDenOutMin=[]  SumDenOutMax=[]  SumNumOutMin=[]  SumNumOutMax=[]  ReciprocalOutMin=[]  ReciprocalOutMax=[]  DivideOutMin=[]  DivideOutMax=[]  TunerSelectOption=Transfer Function Based (PID Tuner App)
  cfblk4 : Sin  TimeSource=Use external signal  SampleTime=0
  cfblk5 : Subsystem
  cfblk6 : Subsystem
  cfblk2 : Outport
  cfblk8 : Outport  Port=2
  cfblk9 : Outport  Port=3
  wires:
  cfblk7/1 -> cfblk2/1, cfblk3/2
  cfblk4/1 -> cfblk5/1(cfblk1)
  cfblk5/1(cfblk2) -> cfblk8/1, cfblk3/1
  cfblk3/1 -> cfblk6/1(cfblk1)
  cfblk6/1(cfblk2) -> cfblk9/1
  cfblk1/1 -> cfblk10/1
  cfblk10/1 -> cfblk4/1

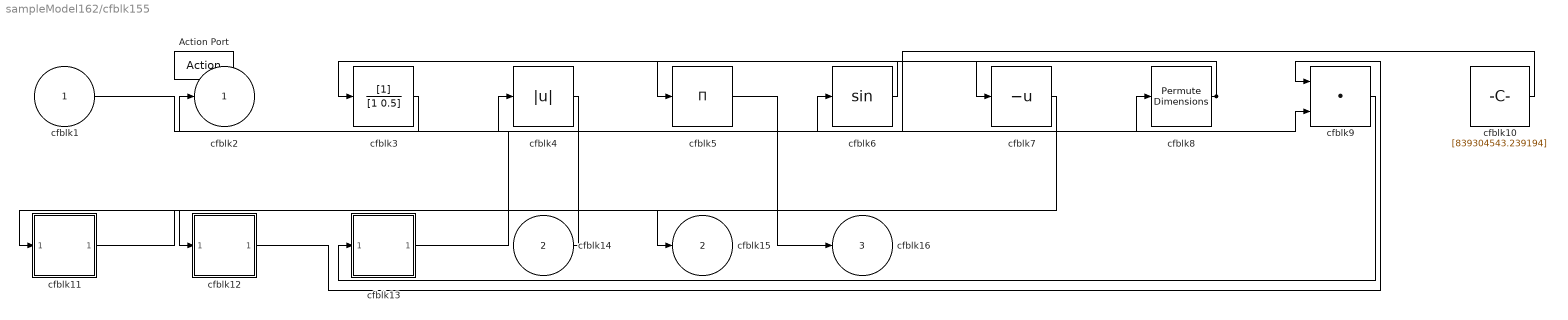
== system sampleModel162/cfblk155 ==
  cfblk1 : Inport
  cfblk14 : Inport  Port=2
  Action Port : ActionPort  ActionType=then
  cfblk10 : Constant  Value=[839304543.239194]  SampleTime=1
  cfblk11 : Subsystem
  cfblk12 : Subsystem
  cfblk13 : Subsystem
  cfblk3 : DiscreteFilter
  cfblk4 : Abs
  cfblk5 : Product  Inputs=*
  cfblk6 : Trigonometry
  cfblk7 : UnaryMinus
  cfblk8 : PermuteDimensions
  cfblk9 : DotProduct  InputSameDT=on  OutDataTypeStr=Inherit: Inherit via internal rule
  cfblk2 : Outport
  cfblk15 : Outport  Port=2
  cfblk16 : Outport  Port=3
  wires:
  cfblk4/1 -> cfblk12/1(cfblk1)
  cfblk3/1 -> cfblk2/1
  cfblk9/1 -> cfblk13/1(cfblk1)
  cfblk11/1(cfblk2) -> cfblk15/1
  cfblk6/1 -> cfblk5/1
  cfblk14/1 -> cfblk4/1
  cfblk5/1 -> cfblk16/1
  cfblk12/1(cfblk2) -> cfblk9/1
  cfblk10/1 -> cfblk6/1
  cfblk13/1(cfblk2) -> cfblk8/1
  cfblk1/1 -> cfblk9/2
  cfblk7/1 -> cfblk11/1(cfblk1)
  cfblk8/1 -> cfblk3/1, cfblk7/1

== system sampleModel162/cfblk156 ==
  cfblk1 : Inport
  cfblk7 : Inport  Port=2
  cfblk8 : Inport  Port=3
  Action Port : ActionPort  ActionType=else
  cfblk10 : Subsystem  TreatAsAtomicUnit=on
  cfblk11 : Delay
  cfblk3 : DiscreteStateSpace  SampleTime=-1
  cfblk4 : simulink/Discrete/Tapped Delay  vinit=0.0  samptime=-1  NumDelays=1  DelayOrder=Oldest  includeCurrent=off
  cfblk5 : MinMax  Inputs=3
  cfblk6 : If  IfExpression=u1 >= 0  SampleTime=1
  cfblk9 : Subsystem  TreatAsAtomicUnit=on
  cfblk2 : Outport
  wires:
  cfblk10/1(cfblk2) -> cfblk2/1
  cfblk7/1 -> cfblk4/1, cfblk10/1(cfblk1)
  cfblk1/1 -> cfblk5/1, cfblk5/3
  cfblk3/1 -> cfblk9/1(cfblk1)
  cfblk5/1 -> cfblk3/1, cfblk10/2(cfblk8)
  cfblk8/1 -> cfblk9/2(cfblk15)
  cfblk4/1 -> cfblk5/2
  cfblk6/1 -> cfblk9/Action
  cfblk6/2 -> cfblk10/Action
  cfblk9/1(cfblk2) -> cfblk11/1
  cfblk11/1 -> cfblk6/1

== system sampleModel162/cfblk157 ==
  cfblk1 : Inport
  Action Port : ActionPort  ActionType=then
  cfblk3 : simulink/Continuous/PID Controller  Controller=PID  TimeDomain=Discrete-time  SampleTime=-1  IntegratorMethod=Forward Euler  FilterMethod=Forward Euler  Form=Parallel  UseFilter=on  ControllerParametersSource=internal  P=1  I=1  D=0  N=100  InitialConditionSource=internal  InitialConditionForIntegrator=0  InitialConditionForFilter=0  ExternalReset=none  LimitOutput=off  UpperSaturationLimit=inf  LowerSaturationLimit=-inf  LinearizeAsGain=off  AntiWindupMode=none  Kb=1  TrackingMode=off  Kt=1  PParamMin=[]  PParamMax=[]  IParamMin=[]  IParamMax=[]  DParamMin=[]  DParamMax=[]  NParamMin=[]  NParamMax=[]  KbParamMin=[]  KbParamMax=[]  KtParamMin=[]  KtParamMax=[]  POutMin=[]  POutMax=[]  IOutMin=[]  IOutMax=[]  DOutMin=[]  DOutMax=[]  NOutMin=[]  NOutMax=[]  KbOutMin=[]  KbOutMax=[]  KtOutMin=[]  KtOutMax=[]  IntegratorOutMin=[]  IntegratorOutMax=[]  FilterOutMin=[]  FilterOutMax=[]  SumOutMin=[]  SumOutMax=[]  SumI1OutMin=[]  SumI1OutMax=[]  SumI2OutMin=[]  SumI2OutMax=[]  SumI3OutMin=[]  SumI3OutMax=[]  SumDOutMin=[]  SumDOutMax=[]  SaturationOutMin=[]  SaturationOutMax=[]  IntegratorContinuousStateAttributes=''  IntegratorStateMustResolveToSignalObject=off  IntegratorRTWStateStorageClass=Auto  FilterContinuousStateAttributes=''  FilterStateMustResolveToSignalObject=off  FilterRTWStateStorageClass=Auto  DifferentiatorICPrevScaledInput=0  DifferentiatorOutMin=[]  DifferentiatorOutMax=[]  FilterDiffOutCoefMin=[]  FilterDiffOutCoefMax=[]  SumDenOutMin=[]  SumDenOutMax=[]  SumNumOutMin=[]  SumNumOutMax=[]  ReciprocalOutMin=[]  ReciprocalOutMax=[]  DivideOutMin=[]  DivideOutMax=[]  TunerSelectOption=Transfer Function Based (PID Tuner App)
  cfblk4 : Constant  Value=[-610127903.820520]  SampleTime=1
  cfblk5 : Constant  Value=[242557199.492521]  SampleTime=1
  cfblk6 : Subsystem
  cfblk7 : Subsystem
  cfblk8 : Subsystem
  cfblk2 : Outport
  wires:
  cfblk3/1 -> cfblk8/1(cfblk1)
  cfblk8/1(cfblk2) -> cfblk6/1(cfblk1)
  cfblk4/1 -> cfblk7/1(cfblk1)
  cfblk1/1 -> cfblk3/1
  cfblk7/1(cfblk2) -> cfblk2/1

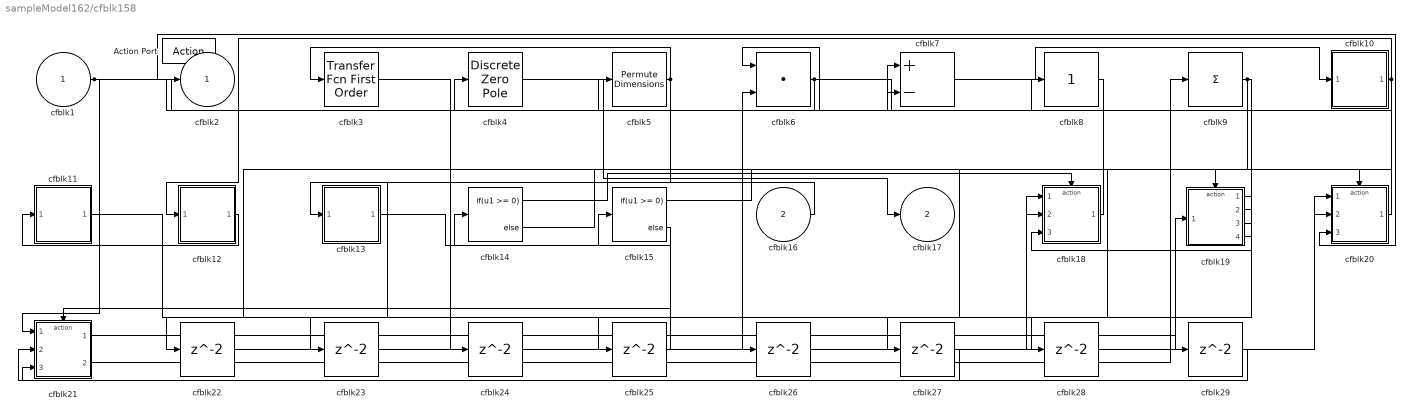
== system sampleModel162/cfblk158 ==
  cfblk1 : Inport
  cfblk16 : Inport  Port=2
  Action Port : ActionPort  ActionType=else
  cfblk10 : Subsystem
  cfblk11 : Subsystem
  cfblk12 : Subsystem
  cfblk13 : Subsystem
  cfblk14 : If  IfExpression=u1 >= 0  SampleTime=1
  cfblk15 : If  IfExpression=u1 >= 0  SampleTime=1
  cfblk18 : Subsystem  TreatAsAtomicUnit=on
  cfblk19 : Subsystem  TreatAsAtomicUnit=on
  cfblk20 : Subsystem  TreatAsAtomicUnit=on
  cfblk21 : Subsystem  TreatAsAtomicUnit=on
  cfblk{22..29} (8 alike) : Delay
  cfblk3 : simulink/Discrete/Transfer Fcn First Order  PoleZ=0.95  ICPrevOutput=0.0  DoSatur=off
      settings: SourceProductName=Simulink
  cfblk4 : DiscreteZeroPole  Poles=[0 0.5]  Gain=1  SampleTime=-1
  cfblk5 : PermuteDimensions
  cfblk6 : DotProduct  InputSameDT=on  OutDataTypeStr=Inherit: Inherit via internal rule
  cfblk7 : Sum  Inputs=+-
  cfblk8 : simulink/Math Operations/Slider Gain  gain=1  low=0  high=2
  cfblk9 : Sum  Inputs=+
  cfblk2 : Outport
  cfblk17 : Outport  Port=2
  wires:
  cfblk21/1(cfblk2) -> cfblk19/1(cfblk1)
  cfblk16/1 -> cfblk13/1(cfblk1)
  cfblk4/1 -> cfblk17/1
  cfblk5/1 -> cfblk3/1, cfblk23/1
  cfblk20/1(cfblk2) -> cfblk6/1
  cfblk9/1 -> cfblk28/1, cfblk29/1
  cfblk10/1(cfblk2) -> cfblk12/1(cfblk1), cfblk27/1
  cfblk7/1 -> cfblk10/1(cfblk1)
  cfblk21/2(cfblk17) -> cfblk9/1
  cfblk13/1(cfblk2) -> cfblk15/1
  cfblk1/1 -> cfblk20/3(cfblk8), cfblk21/1(cfblk1), cfblk7/2
  cfblk19/2(cfblk12) -> cfblk7/1
  cfblk6/1 -> cfblk8/1, cfblk2/1
  cfblk12/1(cfblk2) -> cfblk11/1(cfblk1)
  cfblk18/1(cfblk2) -> cfblk5/1
  cfblk19/3(cfblk13) -> cfblk18/3(cfblk16)
  cfblk19/4(cfblk14) -> cfblk4/1
  cfblk14/1 -> cfblk18/Action
  cfblk14/2 -> cfblk19/Action
  cfblk15/1 -> cfblk20/Action
  cfblk15/2 -> cfblk21/Action
  cfblk8/1 -> cfblk22/1
  cfblk22/1 -> cfblk6/2
  cfblk23/1 -> cfblk20/1(cfblk1)
  cfblk3/1 -> cfblk24/1
  cfblk24/1 -> cfblk18/1(cfblk1)
  cfblk19/1(cfblk2) -> cfblk25/1
  cfblk25/1 -> cfblk14/1
  cfblk11/1(cfblk2) -> cfblk26/1
  cfblk26/1 -> cfblk18/2(cfblk15)
  cfblk27/1 -> cfblk21/2(cfblk15)
  cfblk28/1 -> cfblk20/2(cfblk7)
  cfblk29/1 -> cfblk21/3(cfblk16)

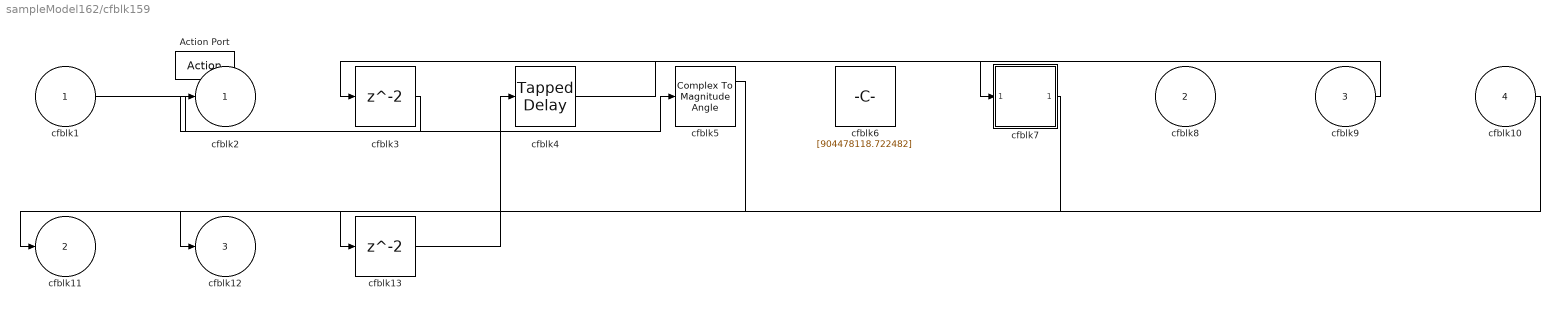
== system sampleModel162/cfblk159 ==
  cfblk1 : Inport
  cfblk8 : Inport  Port=2
  cfblk9 : Inport  Port=3
  cfblk10 : Inport  Port=4
  Action Port : ActionPort  ActionType=then
  cfblk13 : Delay
  cfblk3 : Delay
  cfblk4 : simulink/Discrete/Tapped Delay  vinit=0.0  samptime=-1  NumDelays=1  DelayOrder=Oldest  includeCurrent=off
  cfblk5 : ComplexToMagnitudeAngle
  cfblk6 : Constant  Value=[904478118.722482]  SampleTime=1
  cfblk7 : Subsystem
  cfblk2 : Outport
  cfblk11 : Outport  Port=2
  cfblk12 : Outport  Port=3
  wires:
  cfblk1/1 -> cfblk5/1
  cfblk10/1 -> cfblk11/1
  cfblk9/1 -> cfblk3/1
  cfblk3/1 -> cfblk2/1
  cfblk5/1 -> cfblk12/1
  cfblk4/1 -> cfblk7/1(cfblk1)
  cfblk7/1(cfblk2) -> cfblk13/1
  cfblk13/1 -> cfblk4/1

== system sampleModel162/cfblk160 ==
  cfblk1 : Inport
  cfblk8 : Inport  Port=2
  Action Port : ActionPort  ActionType=else
  cfblk10 : Subsystem  TreatAsAtomicUnit=on
  cfblk11 : Delay
  cfblk12 : Delay
  cfblk3 : simulink/Continuous/PID Controller  Controller=PID  TimeDomain=Discrete-time  SampleTime=-1  IntegratorMethod=Forward Euler  FilterMethod=Forward Euler  Form=Parallel  UseFilter=on  ControllerParametersSource=internal  P=1  I=1  D=0  N=100  InitialConditionSource=internal  InitialConditionForIntegrator=0  InitialConditionForFilter=0  ExternalReset=none  LimitOutput=off  UpperSaturationLimit=inf  LowerSaturationLimit=-inf  LinearizeAsGain=off  AntiWindupMode=none  Kb=1  TrackingMode=off  Kt=1  PParamMin=[]  PParamMax=[]  IParamMin=[]  IParamMax=[]  DParamMin=[]  DParamMax=[]  NParamMin=[]  NParamMax=[]  KbParamMin=[]  KbParamMax=[]  KtParamMin=[]  KtParamMax=[]  POutMin=[]  POutMax=[]  IOutMin=[]  IOutMax=[]  DOutMin=[]  DOutMax=[]  NOutMin=[]  NOutMax=[]  KbOutMin=[]  KbOutMax=[]  KtOutMin=[]  KtOutMax=[]  IntegratorOutMin=[]  IntegratorOutMax=[]  FilterOutMin=[]  FilterOutMax=[]  SumOutMin=[]  SumOutMax=[]  SumI1OutMin=[]  SumI1OutMax=[]  SumI2OutMin=[]  SumI2OutMax=[]  SumI3OutMin=[]  SumI3OutMax=[]  SumDOutMin=[]  SumDOutMax=[]  SaturationOutMin=[]  SaturationOutMax=[]  IntegratorContinuousStateAttributes=''  IntegratorStateMustResolveToSignalObject=off  IntegratorRTWStateStorageClass=Auto  FilterContinuousStateAttributes=''  FilterStateMustResolveToSignalObject=off  FilterRTWStateStorageClass=Auto  DifferentiatorICPrevScaledInput=0  DifferentiatorOutMin=[]  DifferentiatorOutMax=[]  FilterDiffOutCoefMin=[]  FilterDiffOutCoefMax=[]  SumDenOutMin=[]  SumDenOutMax=[]  SumNumOutMin=[]  SumNumOutMax=[]  ReciprocalOutMin=[]  ReciprocalOutMax=[]  DivideOutMin=[]  DivideOutMax=[]  TunerSelectOption=Transfer Function Based (PID Tuner App)
  cfblk4 : DiscreteIntegrator  SampleTime=-1  ICPrevOutput=DiscIntNeverNeededParam  ICPrevScaledInput=DiscIntNeverNeededParam
  cfblk5 : DiscreteTransferFcn
  cfblk6 : Subsystem
  cfblk7 : If  IfExpression=u1 >= 0  SampleTime=1
  cfblk9 : Subsystem  TreatAsAtomicUnit=on
  cfblk2 : Outport
  wires:
  cfblk9/1(cfblk2) -> cfblk4/1
  cfblk5/1 -> cfblk6/1(cfblk1)
  cfblk1/1 -> cfblk5/1
  cfblk3/1 -> cfblk10/1(cfblk1)
  cfblk6/1(cfblk2) -> cfblk2/1
  cfblk10/1(cfblk2) -> cfblk9/1(cfblk1)
  cfblk8/1 -> cfblk9/2(cfblk8)
  cfblk10/2(cfblk16) -> cfblk9/3(cfblk9)
  cfblk10/3(cfblk17) -> cfblk9/4(cfblk10)
  cfblk7/1 -> cfblk9/Action
  cfblk7/2 -> cfblk10/Action
  cfblk4/1 -> cfblk11/1
  cfblk11/1 -> cfblk3/1
  cfblk9/2(cfblk11) -> cfblk12/1
  cfblk12/1 -> cfblk7/1

== system sampleModel162/cfblk161 ==
  cfblk1 : Inport
  Action Port : ActionPort  ActionType=then
  cfblk3 : simulink/Discrete/Transfer Fcn First Order  PoleZ=0.95  ICPrevOutput=0.0  DoSatur=off
      settings: SourceProductName=Simulink
  cfblk4 : Sum  Inputs=+-
  cfblk5 : Subsystem
  cfblk6 : Subsystem
  cfblk7 : Subsystem
  cfblk9 : Delay
  cfblk2 : Outport
  cfblk8 : Outport  Port=2
  wires:
  cfblk4/1 -> cfblk8/1
  cfblk5/1(cfblk2) -> cfblk4/1, cfblk9/1
  cfblk1/1 -> cfblk2/1
  cfblk6/1(cfblk2) -> cfblk5/1(cfblk1)
  cfblk7/1(cfblk2) -> cfblk6/1(cfblk1)
  cfblk3/1 -> cfblk7/1(cfblk1), cfblk4/2
  cfblk9/1 -> cfblk3/1

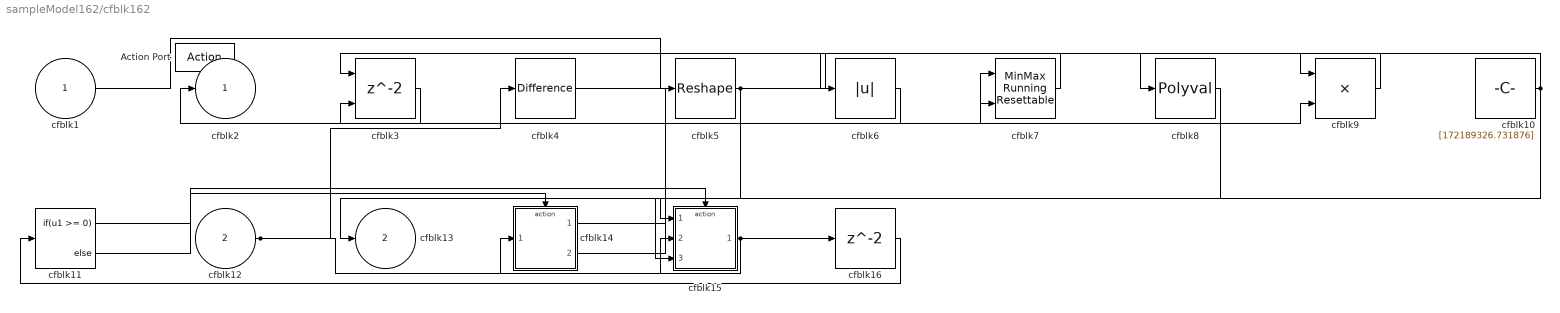
== system sampleModel162/cfblk162 ==
  cfblk1 : Inport
  cfblk12 : Inport  Port=2
  Action Port : ActionPort  ActionType=else
  cfblk10 : Constant  Value=[172189326.731876]  SampleTime=1
  cfblk11 : If  IfExpression=u1 >= 0  SampleTime=1
  cfblk14 : Subsystem  TreatAsAtomicUnit=on
  cfblk15 : Subsystem  TreatAsAtomicUnit=on
  cfblk16 : Delay
  cfblk3 : Delay  ShowEnablePort=on
      settings: InputPortMap=u0,e6
  cfblk4 : simulink/Discrete/Difference  ICPrevInput=0.0  OutMin=[]  OutMax=[]  OutDataTypeStr=Inherit: Inherit via back propagation  OutDataType=fixdt(1, 16)  OutScaling=2^-10  DoSatur=off
  cfblk5 : Reshape
  cfblk6 : Abs
  cfblk7 : simulink/Math Operations/MinMax Running Resettable  Function=min  vinit=0.0
  cfblk8 : Polyval  Coefs=[ +2.081618890e-019, -1.441693666e-014, +4.719686976e-010, -8.536869453e-006, +1.621573104e-001, -8.087801117e+001 ]
  cfblk9 : Product  Inputs=**
  cfblk2 : Outport
  cfblk13 : Outport  Port=2
  wires:
  cfblk8/1 -> cfblk13/1
  cfblk5/1 -> cfblk9/1, cfblk15/1(cfblk1)
  cfblk10/1 -> cfblk8/1, cfblk15/3(cfblk8)
  cfblk3/1 -> cfblk2/1
  cfblk4/1 -> cfblk7/1
  cfblk15/1(cfblk2) -> cfblk14/1(cfblk1), cfblk16/1
  cfblk12/1 -> cfblk4/1, cfblk15/2(cfblk7)
  cfblk1/1 -> cfblk5/1
  cfblk7/1 -> cfblk3/1
  cfblk6/1 -> cfblk3/2
  cfblk14/1(cfblk2) -> cfblk7/2
  cfblk9/1 -> cfblk6/1
  cfblk14/2(cfblk15) -> cfblk9/2
  cfblk11/1 -> cfblk14/Action
  cfblk11/2 -> cfblk15/Action
  cfblk16/1 -> cfblk11/1

== system sampleModel162/cfblk163 ==
  cfblk1 : Inport
  Action Port : ActionPort  ActionType=then
  cfblk3 : simulink/Discrete/Tapped Delay  vinit=0.0  samptime=-1  NumDelays=1  DelayOrder=Oldest  includeCurrent=off
  cfblk4 : UnaryMinus
  cfblk5 : Subsystem
  cfblk2 : Outport
  cfblk6 : Outport  Port=2
  cfblk7 : Outport  Port=3
  wires:
  cfblk1/1 -> cfblk5/1(cfblk1), cfblk2/1
  cfblk4/1 -> cfblk3/1
  cfblk3/1 -> cfblk7/1, cfblk6/1
  cfblk5/1(cfblk2) -> cfblk4/1

== system sampleModel162/cfblk164 ==
  cfblk1 : Inport
  cfblk10 : Inport  Port=2
  Action Port : ActionPort  ActionType=else
  cfblk13 : Delay
  cfblk3 : DiscreteIntegrator  SampleTime=-1  ICPrevOutput=DiscIntNeverNeededParam  ICPrevScaledInput=DiscIntNeverNeededParam
  cfblk4 : Delay
  cfblk5 : simulink/Discrete/Transfer Fcn Lead or Lag  PoleZ=0.95  ZeroZ=0.75  ICPrevOutput=0.0  ICPrevInput=0.0  DoSatur=off
      settings: SourceProductName=Simulink  SourceProductBaseCode=SL
  cfblk6 : Subsystem
  cfblk7 : Subsystem
  cfblk8 : Subsystem
  cfblk9 : Subsystem
  cfblk2 : Outport
  cfblk11 : Outport  Port=2
  cfblk12 : Outport  Port=3
  wires:
  cfblk7/1(cfblk2) -> cfblk12/1
  cfblk1/1 -> cfblk9/1(cfblk1)
  cfblk3/1 -> cfblk7/1(cfblk1)
  cfblk5/1 -> cfblk11/1
  cfblk8/1(cfblk2) -> cfblk5/1, cfblk3/1
  cfblk9/1(cfblk2) -> cfblk8/1(cfblk1)
  cfblk4/1 -> cfblk6/1(cfblk1)
  cfblk10/1 -> cfblk2/1
  cfblk6/1(cfblk2) -> cfblk13/1
  cfblk13/1 -> cfblk4/1

== system sampleModel162/cfblk151/cfblk10 ==
  cfblk1 : Inport
  cfblk2 : Outport
  wires:
  cfblk1/1 -> cfblk2/1

== system sampleModel162/cfblk151/cfblk11 ==
  cfblk1 : Inport
  cfblk2 : Outport
  wires:
  cfblk1/1 -> cfblk2/1

== system sampleModel162/cfblk151/cfblk12 ==
  cfblk1 : Inport
  cfblk2 : Outport
  wires:
  cfblk1/1 -> cfblk2/1

== system sampleModel162/cfblk151/cfblk13 ==
  cfblk1 : Inport
  cfblk2 : Outport
  wires:
  cfblk1/1 -> cfblk2/1

== system sampleModel162/cfblk152/cfblk6 ==
  cfblk1 : Inport
  cfblk2 : Outport
  wires:
  cfblk1/1 -> cfblk2/1

== system sampleModel162/cfblk152/cfblk7 ==
  cfblk1 : Inport
  cfblk2 : Outport
  wires:
  cfblk1/1 -> cfblk2/1

== system sampleModel162/cfblk153/cfblk8 ==
  cfblk1 : Inport
  cfblk2 : Outport
  wires:
  cfblk1/1 -> cfblk2/1

== system sampleModel162/cfblk153/cfblk9 ==
  cfblk1 : Inport
  cfblk2 : Outport
  wires:
  cfblk1/1 -> cfblk2/1

== system sampleModel162/cfblk154/cfblk5 ==
  cfblk1 : Inport
  cfblk2 : Outport
  wires:
  cfblk1/1 -> cfblk2/1

== system sampleModel162/cfblk154/cfblk6 ==
  cfblk1 : Inport
  cfblk2 : Outport
  wires:
  cfblk1/1 -> cfblk2/1

== system sampleModel162/cfblk155/cfblk11 ==
  cfblk1 : Inport
  cfblk2 : Outport
  wires:
  cfblk1/1 -> cfblk2/1

== system sampleModel162/cfblk155/cfblk12 ==
  cfblk1 : Inport
  cfblk2 : Outport
  wires:
  cfblk1/1 -> cfblk2/1

== system sampleModel162/cfblk155/cfblk13 ==
  cfblk1 : Inport
  cfblk2 : Outport
  wires:
  cfblk1/1 -> cfblk2/1

== system sampleModel162/cfblk156/cfblk10 ==
  cfblk1 : Inport
  cfblk8 : Inport  Port=2
  Action Port : ActionPort  ActionType=else
  cfblk3 : simulink/Discrete/Transfer Fcn Real Zero  ZeroZ=0.75  ICPrevInput=0.0  DoSatur=off
      settings: SourceProductName=Simulink  SourceProductBaseCode=SL
  cfblk4 : Delay  DelayLengthSource=Input port
      settings: InputPortMap=u0,p1
  cfblk5 : Sum  Inputs=+-
  cfblk6 : Product
  cfblk7 : Subsystem
  cfblk9 : Delay
  cfblk2 : Outport
  wires:
  cfblk4/1 -> cfblk2/1
  cfblk6/1 -> cfblk7/1(cfblk1)
  cfblk1/1 -> cfblk5/2
  cfblk8/1 -> cfblk3/1, cfblk4/2, cfblk6/2
  cfblk3/1 -> cfblk4/1
  cfblk5/1 -> cfblk6/1
  cfblk7/1(cfblk2) -> cfblk9/1
  cfblk9/1 -> cfblk5/1
